simulink model "AnalogNeuronSimpleTest"  (Simulink 10.2)
settings: Solver=ode45  StartTime=0.0  StopTime=1  RelTol=1e-3  EnableMultiTasking=on
libraries: NeuroModelerLibrary x3
settings Model: Creator=user  LastModifiedBy=Bakhshiev
settings DataIOCC: LimitDataPoints=on
settings OptimizationCC: ExpressionDepthLimit=2147483647
settings DebuggingCC: SolverPrmCheckMsg=warning  StateNameClashWarn=warning
settings ConfigComp: CovSFcnEnable=off

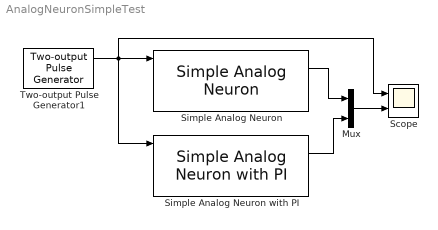
== system AnalogNeuronSimpleTest ==
  Mux : Mux  Inputs=2
  Scope : Scope  NumInputPorts=2
  Simple Analog Neuron : NeuroModelerLibrary/Analog Simple Cells/Simple Analog Neuron  SystemSampleTime=-1  VariantActivationTime=update diagram  Latency=0  AutoFrameSizeCalculation=off
  Simple Analog Neuron with PI : NeuroModelerLibrary/Analog Simple Cells/Simple Analog Neuron with PI  SystemSampleTime=-1  VariantActivationTime=update diagram  Latency=0  AutoFrameSizeCalculation=off
  Two-output Pulse Generator1 : NeuroModelerLibrary/Support/Two-output Pulse Generator  A=1  P1=200  P2=200  PW=1  ST=0.001  OOn1=0.3  OOff1=0.6  OOn2=1.1  OOff2=1.2
  wires:
  Two-output Pulse Generator1/1 -> Simple Analog Neuron with PI/1, Simple Analog Neuron/1, Scope/1
  Mux/1 -> Scope/2
  Simple Analog Neuron/1 -> Mux/1
  Simple Analog Neuron with PI/1 -> Mux/2
